simulink model "xinshi"  (R2022b)
settings: Solver=VariableStepAuto  StartTime=0.0  StopTime=100  RelTol=1e-3
settings Model: Creator=22601  LastModifiedBy=22601

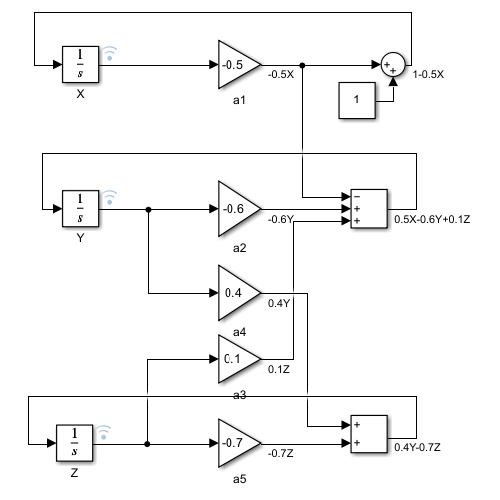
[thumbnail: Simulink's stored preview of the top-level diagram]
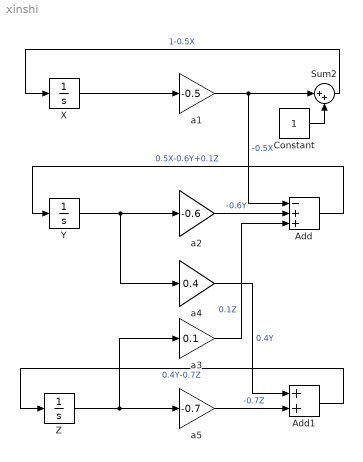
== system xinshi ==
  Add : Sum  Inputs=-++
  Add1 : Sum
  Constant : Constant
  Sum2 : Sum  Inputs=|++
  X : Integrator
  Y : Integrator  InitialCondition=10
  Z : Integrator
  a1 : Gain  Gain=-0.5
  a2 : Gain  Gain=-0.6
  a3 : Gain  Gain=0.1
  a4 : Gain  Gain=0.4
  a5 : Gain  Gain=-0.7
  wires:
  X/1 -> a1/1
  a1/1 -> Add/1, Sum2/1  "-0.5X"
  Constant/1 -> Sum2/2
  Sum2/1 -> X/1  "1-0.5X"
  Y/1 -> a4/1, a2/1
  a2/1 -> Add/2  "-0.6Y"
  Z/1 -> a3/1, a5/1
  a5/1 -> Add1/2  "-0.7Z"
  a4/1 -> Add1/1  "0.4Y"
  Add1/1 -> Z/1  "0.4Y-0.7Z"
  a3/1 -> Add/3  "0.1Z"
  Add/1 -> Y/1  "0.5X-0.6Y+0.1Z"
